simulink model "Model_14Bus_Microgrid_paper_Latam"  (R2022b)
settings: Solver=VariableStepAuto  StartTime=0.0  StopTime=0.5  MaxStep=1e-2  RelTol=1e-3
InitFcn:
  | Set_parameters_R2018
StopFcn:
  | %Save_Data;
  | %Graphics_mod;
values from neighbouring files (symbols this model uses):
  Clink = Ceq*2    (= 0.217013888889)    [Set_parameters.m]
  dis1 = 0.15    [Set_parameters.m]
  dis10 = 6    [Set_parameters.m]
  dis11 = 3    [Set_parameters.m]
  dis12 = 6    [Set_parameters.m]
  dis13 = 3    [Set_parameters.m]
  dis14 = 2    [Set_parameters.m]
  dis2 = 0.2    [Set_parameters.m]
  dis3 = 0.15    [Set_parameters.m]
  dis4 = 0.4    [Set_parameters.m]
  dis5 = 0.4    [Set_parameters.m]
  dis6 = 0.4    [Set_parameters.m]
  dis7 = 0.1    [Set_parameters.m]
  dis8 = 2    [Set_parameters.m]
  dis9 = 6    [Set_parameters.m]
  Fc = 33 * Fnom    (= 1980)    [Set_parameters.m]
  Fnom = 60    [Set_parameters.m]
  Increment_MPPT = 0.01    [Set_parameters.m]
  Ki_Ireg = 20    [Set_parameters.m]
  Ki_VDCreg = 400    [Set_parameters.m]
  Kp_Ireg = 0.3    [Set_parameters.m]
  Kp_VDCreg = 2    [Set_parameters.m]
  LimitL_Ireg = -1.5    [Set_parameters.m]
  LimitL_VDCreg = -1.5    [Set_parameters.m]
  Limits_MPPT = [ 583 357 ]    [Set_parameters.m]
  LimitU_Ireg = 1.5    [Set_parameters.m]
  LimitU_VDCreg = 1.5    [Set_parameters.m]
  P_Load_2 = S_Load_2* PF_Load_2    (= 36000)    [Set_parameters.m]
  P_Load_3 = S_Load_3* PF_Load_3    (= 25500)    [Set_parameters.m]
  Pnom = 1e6    (= 1000000)    [Set_parameters.m]
  Pnom_T1 = 1.5e6    (= 1500000)    [Set_parameters.m]
  Pnom_T2 = 1.5e6    (= 1500000)    [Set_parameters.m]
  Pnom_T3 = 4e6    (= 4000000)    [Set_parameters.m]
  Pnom_xfo = Pnom    (= 1000000)    [Set_parameters.m]
  Ql_Load_2 = S_Load_2 * sin(acos(PF_Load_2))    [Set_parameters.m]
  Ql_Load_3 = S_Load_3 * sin(acos(PF_Load_3))    [Set_parameters.m]
  R_Load_9 = (Vnom_prim * 1.35)^2 / P_Load_9    (= 1084.6153125)    [Set_parameters.m]
  R_Load_DC = Vnom_DC^2/ P_Load_DC    (= 45)    [Set_parameters.m]
  Rl = 0.394    [Set_parameters.m]
  Rls = 0.198    [Set_parameters.m]
  Ts = Ts_Power    (= 5.05050505051e-06)    [Set_parameters.m]
  Ts_Control = 10*Ts_Power    (= 5.05050505051e-05)    [Set_parameters.m]
  Ts_Power = 1/(33*Fnom)/100    (= 5.05050505051e-06)    [Set_parameters.m]
  V1_LL_T3 = 69e3    (= 69000)    [Set_parameters.m]
  Vf = 0    [Set_parameters.m]
  Vfd = 0    [Set_parameters.m]
  Vnom_dc = 480    [Set_parameters.m]
  Vnom_Diesel = 2.4e3    (= 2400)    [Set_parameters.m]
  Vnom_prim = 13.8e3    (= 13800)    [Set_parameters.m]
  Vnom_sec = 220    [Set_parameters.m]
  Vnom_ter_AC_DC = 150    [Set_parameters.m]
  Xl = 0.1168    [Set_parameters.m]
  Xls = 0.1089    [Set_parameters.m]
undefined symbols (not defined in the file or in its folder): D1, Delta, DiscIntNeverNeededParam, Hydride, Ion, level, Lithium, max_min, Metal, Nickel, RL, RLff, sigbuilder_block
libraries: spsRMSLib x73, powerlib_extras x53, spsCurrentMeasurementLib x47, spsTHDLib x26, spsThreePhaseVIMeasurementLib x25, spsVoltageMeasurementLib x23, spsSeriesRLCBranchLib x21, spsThreePhaseSeriesRLCBranchLib x21, spsIGBTDiodeLib x15, spsThreePhaseBreakerLib x14, spsPowerLib x14, spsThreePhaseTransformerTwoWindingsLib x12
(part 1 of 10)
settings Model: Creator=Leony  LastModifiedBy=christian
settings SolverCC: ZeroCrossAlgorithm=Adaptive  AlgebraicLoopSolver=TrustRegion  SolverResetMethod=Robust
settings DataIOCC: LimitDataPoints=on  SaveFormat=Array  ReturnWorkspaceOutputs=off
settings OptimizationCC: LifeSpan=inf  AccelVerboseBuild=on
settings DebuggingCC: AlgebraicLoopMsg=none  UnderspecifiedInitializationDetection=Classic  MergeDetectMultiDrivingBlocksExec=none  IgnoredZcDiagnostic=none  SolverPrmCheckMsg=warning  AllowSymbolicDim=off  SFUnexpectedBacktrackingDiag=warning  SFNoUnconditionalDefaultTransitionDiag=warning  SFExecutionAtInitializationDiag=none  SFMachineParentedDataDiag=warning  ArithmeticOperatorsInVariantConditions=warning
settings HardwareCC: ProdBitPerPointer=32  ProdBitPerSizeT=32  ProdBitPerPtrDiffT=32  ProdLargestAtomicFloat=None  ProdIntDivRoundTo=Undefined  ProdEndianess=Unspecified  ProdWordSize=32  ProdHWDeviceType=32-bit Generic
settings ModelReferenceCC: EnableRefExpFcnMdlSchedulingChecks=on  PropagateSignalLabelsOutOfModel=off
settings SFSimCC: SimUseLocalCustomCode=off  CustomCodeUndefinedFunction=UseInterfaceOnly
settings RTWCC: RTWUseLocalCustomCode=off  DLArmComputeVersion=19.05
settings CodeAppCC: StateflowObjectComments=on
settings GRTTargetCC: TargetLangStandard=C89/C90 (ANSI)
settings ConfigComp: CovMetricSettings=dw  CovSaveCumulativeToWorkspaceVar=on  CovSaveSingleToWorkspaceVar=on  CovExternalEMLEnable=off
settings SimscapeCC: SimscapeNormalizeSystem=off

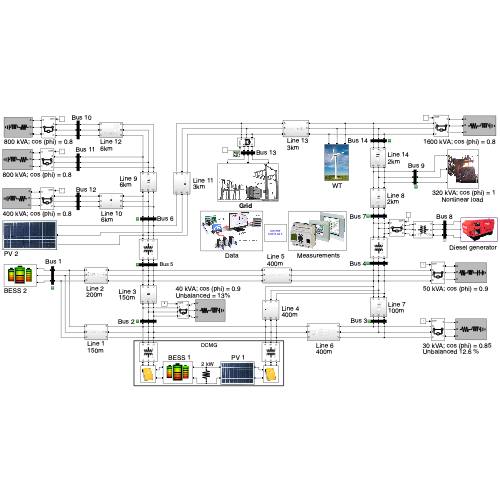
[thumbnail: Simulink's stored preview of the top-level diagram]
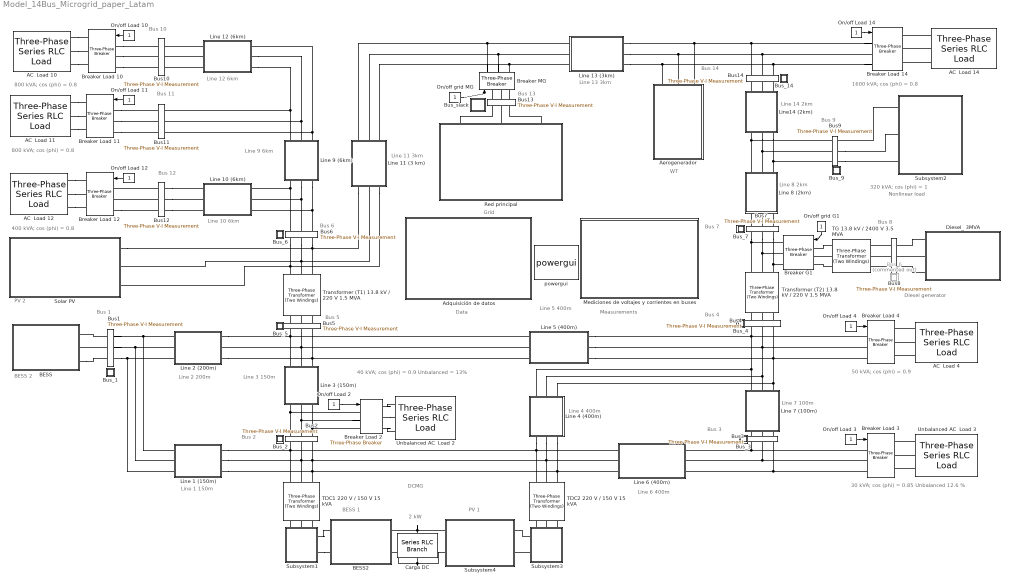
== system Model_14Bus_Microgrid_paper_Latam ==
  note: 1600 kVA; cos (phi) = 0.8
  note: 800 kVA; cos (phi) = 0.8
  note: 400 kVA; cos (phi) = 0.8
  note: 800 kVA; cos (phi) = 0.8
  note: 50 kVA; cos (phi) = 0.9
  note: 40 kVA; cos (phi) = 0.9
      | Unbalanced = 13%
  note: 2 kW
  note: 30 kVA; cos (phi) = 0.85
      | Unbalanced 12.6 %
  note: 320 kVA; cos (phi) = 1
  note: Diesel generator
  note: Line 7
      | 100m
  note: Bus 3
  note: Bus 2
  note: Bus 1
  note: Bus 5
  note: Bus 4
  note: Bus 6
  note: Bus 7
  note: Bus 9
  note: Bus 14
  note: Bus 8
  note: Line 8
      | 2km
  note: WT
  note: Line 13
      | 3km
  note: Line 14
      | 2km
  note: Bus 13
  note: Line 11
      | 3km
  note: Line 9
      | 6km
  note: Line 10
      | 6km
  note: Bus 12
  note: Bus 11
  note: Bus 10
  note: Line 12
      | 6km
  note: PV 2
  note: BESS 2
  note: Line 2
      | 200m
  note: Line 3
      | 150m
  note: Line 1
      | 150m
  note: Line 6
      | 400m
  note: Line 4
      | 400m
  note: Line 5
      | 400m
  note: BESS 1
  note: PV 1
  note: Grid
  note: Data
  note: Measurements
  note: Nonlinear load
  note: DCMG
  " Bus13" : spsThreePhaseVIMeasurementLib/Three-Phase V-I Measurement  VoltageMeasurement=phase-to-ground  SetLabelV=on  LabelV=Vabc_Sec  Vpu=off  VpuLL=off  CurrentMeasurement=yes  SetLabelI=on  LabelI=Iabc_Sec  Ipu=off  Pbase=100e6  Vbase=500e3  OutputType=Complex  PhasorSimulation=off  PSBequivalent=0
  AC  Load 10 : spsThreePhaseSeriesRLCLoadLib/Three-Phase Series RLC Load  LConnTagsString=A|B|C  Configuration=Y (grounded)  NominalVoltage=Vnom_prim  Vabc=[1e3 1e3 1e3]  Vabcp=[1e3 1e3 1e3]  NominalFrequency=Fnom  UnbalancedPower=off  ActivePower=P_Load_10  InductivePower=Ql_Load_10  CapacitivePower=0  Pabc=[10e3 9e3 11e3]  QLabc=[100 90 110]  QCabc=[100 90 110]  Pabcp=[10e3 9e3 11e3]  QLabcp=[100 90 110]  QCabcp=[100 90 110]  Measurements=None  LoadType=constant Z
  AC  Load 11 : spsThreePhaseSeriesRLCLoadLib/Three-Phase Series RLC Load  LConnTagsString=A|B|C  Configuration=Y (grounded)  NominalVoltage=Vnom_prim  Vabc=[1e3 1e3 1e3]  Vabcp=[1e3 1e3 1e3]  NominalFrequency=Fnom  UnbalancedPower=off  ActivePower=P_Load_11  InductivePower=Ql_Load_11  CapacitivePower=0  Pabc=[10e3 9e3 11e3]  QLabc=[100 90 110]  QCabc=[100 90 110]  Pabcp=[10e3 9e3 11e3]  QLabcp=[100 90 110]  QCabcp=[100 90 110]  Measurements=None  LoadType=constant Z
  AC  Load 12 : spsThreePhaseSeriesRLCLoadLib/Three-Phase Series RLC Load  LConnTagsString=A|B|C  Configuration=Y (grounded)  NominalVoltage=Vnom_prim  Vabc=[1e3 1e3 1e3]  Vabcp=[1e3 1e3 1e3]  NominalFrequency=Fnom  UnbalancedPower=off  ActivePower=P_Load_12  InductivePower=Ql_Load_12  CapacitivePower=0  Pabc=[10e3 9e3 11e3]  QLabc=[100 90 110]  QCabc=[100 90 110]  Pabcp=[10e3 9e3 11e3]  QLabcp=[100 90 110]  QCabcp=[100 90 110]  Measurements=None  LoadType=constant Z
  AC  Load 14 : spsThreePhaseSeriesRLCLoadLib/Three-Phase Series RLC Load  LConnTagsString=A|B|C  Configuration=Y (grounded)  NominalVoltage=Vnom_prim  Vabc=[1e3 1e3 1e3]  Vabcp=[1e3 1e3 1e3]  NominalFrequency=Fnom  UnbalancedPower=off  ActivePower=P_Load_14  InductivePower=Ql_Load_14  CapacitivePower=0  Pabc=[10e3 9e3 11e3]  QLabc=[100 90 110]  QCabc=[100 90 110]  Pabcp=[10e3 9e3 11e3]  QLabcp=[100 90 110]  QCabcp=[100 90 110]  Measurements=None  LoadType=constant Z
  AC  Load 4 : spsThreePhaseSeriesRLCLoadLib/Three-Phase Series RLC Load  LConnTagsString=A|B|C  Configuration=Y (grounded)  NominalVoltage=Vnom_sec  Vabc=[1e3 1e3 1e3]  Vabcp=[1e3 1e3 1e3]  NominalFrequency=Fnom  UnbalancedPower=on  ActivePower=P_Load_4  InductivePower=Ql_Load_4  CapacitivePower=0  Pabc=[10e3 9e3 11e3]  QLabc=[100 90 110]  QCabc=[100 90 110]  Pabcp=[10e3 9e3 11e3]  QLabcp=[100 90 110]  QCabcp=[100 90 110]  Measurements=None  LoadType=constant Z
  Adquisición de datos : Subsystem
      mask Display: image('/Users/christian/Documents/MATLAB/doctorado/4 conectada a la red con generador diesel, con generacion renovanble (fv)-con almacenamiento varios scope/Icons/SCADA.png'); % Use "Edit Image" on toolstrip to change.
  Aerogenerador : Subsystem
      settings: PortSchema="{\"entries\":[{\"content\":{\"sides\":[{\"content\":{\"connectorIds\":[]},\"type\":\"ConnectorPlacement.EquallySpacedRectSide\",\"uuid\":\"8edb4f72-423a-4d55-86f9-948b81889929\"},{\"content\":{\"connectorIds\":[],\"side\":\"RIGHT\"},\"type\":\"ConnectorPlacement.EquallySpacedRectSide\",\"uuid\":\"0da3ab69-be4e-4974-81d1-ba53ed348584\"},{\"content\":{\"connectorIds\":[\"LConn1\",\"LConn2\",\"LConn3\"],\"side\":\"TOP\"},\"type\":\"ConnectorPlacement.EquallySpacedRectSide\",\"uuid\":\"4000a557-50d9-4ea4-8b49-02707370a143\"}]},\"type\":\"ConnectorPlacement.EquallySpacedConnector\",\"uuid\":\"8a6f3a0d-9558-4751-993e-b03b26ac4eed\"}],\"packageUris\":[\"http://schema.mathworks.com/mf0/Connector/R2020b\"],\"version\":\"1.0\"}"
      mask Display: image('/Users/christian/Documents/MATLAB/doctorado/4 conectada a la red con generador diesel, con generacion renovanble (fv)-con almacenamiento varios scope/Icons/aerogenerador.jpeg'); % Use "Edit Image" on toolstrip to change.
  BESS : Subsystem
      mask Display: image('/Users/christian/Documents/MATLAB/doctorado/4 conectada a la red con generador diesel, con generacion renovanble (fv)-con almacenamiento varios scope/Icons/Battery Energy Storage System (BESS).png'); % Use "Edit Image" on toolstrip to change.
  BESS2 : Subsystem
      mask Display: image('/Users/christian/Documents/MATLAB/doctorado/4 conectada a la red con generador diesel, con generacion renovanble (fv)-con almacenamiento varios scope/Icons/Battery Energy Storage System (BESS).png'); % Use "Edit Image" on toolstrip to change.
  Breaker G1 : spsThreePhaseBreakerLib/Three-Phase Breaker  InitialState=closed  SwitchA=on  SwitchB=on  SwitchC=on  SwitchTimes="[4/60  10/60]"  External=on  BreakerResistance=0.001  SnubberResistance=1e6  SnubberCapacitance=inf  Measurements=None
  Breaker Load {2..4,10..12,14} (7 alike) : spsThreePhaseBreakerLib/Three-Phase Breaker  InitialState=closed  SwitchA=on  SwitchB=on  SwitchC=on  SwitchTimes="[4/60  10/60]"  External=on  BreakerResistance=0.001  SnubberResistance=1e6  SnubberCapacitance=inf  Measurements=None
  Breaker MG : spsThreePhaseBreakerLib/Three-Phase Breaker  InitialState=closed  SwitchA=on  SwitchB=on  SwitchC=on  SwitchTimes="[4/60  10/60]"  External=on  BreakerResistance=0.001  SnubberResistance=1e6  SnubberCapacitance=inf  Measurements=None
  Bus1 : spsThreePhaseVIMeasurementLib/Three-Phase V-I Measurement  VoltageMeasurement=phase-to-ground  SetLabelV=on  LabelV=VabcLL_Bus_1  Vpu=off  VpuLL=off  CurrentMeasurement=yes  SetLabelI=on  LabelI=IabcLL_Bus_1  Ipu=off  Pbase=100e6  Vbase=380/sqrt(2)  OutputType=Complex  PhasorSimulation=off  PSBequivalent=0
  Bus10 : spsThreePhaseVIMeasurementLib/Three-Phase V-I Measurement  VoltageMeasurement=phase-to-ground  SetLabelV=on  LabelV=VabcLL_Bus_10  Vpu=off  VpuLL=off  CurrentMeasurement=yes  SetLabelI=on  LabelI=IabcLL_Bus_10  Ipu=off  Pbase=100e6  Vbase=25e3/sqrt(2)  OutputType=Complex  PhasorSimulation=off  PSBequivalent=0
  Bus11 : spsThreePhaseVIMeasurementLib/Three-Phase V-I Measurement  VoltageMeasurement=phase-to-ground  SetLabelV=on  LabelV=VabcLL_Bus_11  Vpu=off  VpuLL=off  CurrentMeasurement=yes  SetLabelI=on  LabelI=IabcLL_Bus_11  Ipu=off  Pbase=100e6  Vbase=25e3/sqrt(2)  OutputType=Complex  PhasorSimulation=off  PSBequivalent=0
  Bus12 : spsThreePhaseVIMeasurementLib/Three-Phase V-I Measurement  VoltageMeasurement=phase-to-ground  SetLabelV=on  LabelV=VabcLL_Bus_12  Vpu=off  VpuLL=off  CurrentMeasurement=yes  SetLabelI=on  LabelI=IabcLL_Bus_12  Ipu=off  Pbase=100e6  Vbase=25e3  OutputType=Complex  PhasorSimulation=off  PSBequivalent=0
  Bus14 : spsThreePhaseVIMeasurementLib/Three-Phase V-I Measurement  VoltageMeasurement=phase-to-ground  SetLabelV=on  LabelV=VabcLL_Bus_14  Vpu=off  VpuLL=off  CurrentMeasurement=yes  SetLabelI=on  LabelI=IabcLL_Bus_14  Ipu=off  Pbase=100e6  Vbase=25e3/sqrt(2)  OutputType=Complex  PhasorSimulation=off  PSBequivalent=0
  Bus2 : spsThreePhaseVIMeasurementLib/Three-Phase V-I Measurement  VoltageMeasurement=phase-to-ground  SetLabelV=on  LabelV=VabcLL_Bus_2  Vpu=off  VpuLL=off  CurrentMeasurement=yes  SetLabelI=on  LabelI=IabcLL_Bus_2  Ipu=off  Pbase=100e6  Vbase=380/sqrt(2)  OutputType=Complex  PhasorSimulation=off  PSBequivalent=0
  Bus3 : spsThreePhaseVIMeasurementLib/Three-Phase V-I Measurement  VoltageMeasurement=phase-to-ground  SetLabelV=on  LabelV=VabcLL_Bus_3  Vpu=off  VpuLL=off  CurrentMeasurement=yes  SetLabelI=on  LabelI=IabcLL_Bus_3  Ipu=off  Pbase=100e6  Vbase=500e3  OutputType=Complex  PhasorSimulation=off  PSBequivalent=0
  Bus4 : spsThreePhaseVIMeasurementLib/Three-Phase V-I Measurement  VoltageMeasurement=phase-to-ground  SetLabelV=on  LabelV=VabcLL_Bus_4  Vpu=off  VpuLL=off  CurrentMeasurement=yes  SetLabelI=on  LabelI=IabcLL_Bus_4  Ipu=off  Pbase=100e6  Vbase=380/sqrt(2)  OutputType=Complex  PhasorSimulation=off  PSBequivalent=0
  Bus5 : spsThreePhaseVIMeasurementLib/Three-Phase V-I Measurement  VoltageMeasurement=phase-to-ground  SetLabelV=on  LabelV=VabcLL_Bus_5  Vpu=off  VpuLL=off  CurrentMeasurement=yes  SetLabelI=on  LabelI=IabcLL_Bus_5  Ipu=off  Pbase=100e6  Vbase=380/sqrt(2)  OutputType=Complex  PhasorSimulation=off  PSBequivalent=0
  Bus6 : spsThreePhaseVIMeasurementLib/Three-Phase V-I Measurement  VoltageMeasurement=phase-to-ground  SetLabelV=on  LabelV=VabcLL_Bus_6  Vpu=off  VpuLL=off  CurrentMeasurement=yes  SetLabelI=on  LabelI=IabcLL_Bus_6  Ipu=off  Pbase=100e6  Vbase=25e3/sqrt (2)  OutputType=Complex  PhasorSimulation=off  PSBequivalent=0
  Bus7_ : spsThreePhaseVIMeasurementLib/Three-Phase V-I Measurement  VoltageMeasurement=phase-to-ground  SetLabelV=on  LabelV=VabcLL_Bus_7  Vpu=off  VpuLL=off  CurrentMeasurement=yes  SetLabelI=on  LabelI=IabcLL_Bus_7  Ipu=off  Pbase=100e6  Vbase=25e3/sqrt(2)  OutputType=Complex  PhasorSimulation=off  PSBequivalent=0
  Bus8 : spsThreePhaseVIMeasurementLib/Three-Phase V-I Measurement  VoltageMeasurement=phase-to-ground  SetLabelV=on  LabelV=VabcLL_Bus_8  Vpu=off  VpuLL=off  CurrentMeasurement=yes  SetLabelI=on  LabelI=IabcLL_Bus_8  Ipu=off  Pbase=100e6  Vbase=25e3/sqrt(2)  OutputType=Complex  PhasorSimulation=off  PSBequivalent=0
  Bus9 : spsThreePhaseVIMeasurementLib/Three-Phase V-I Measurement  VoltageMeasurement=phase-to-ground  SetLabelV=on  LabelV=VabcLL_Bus_9  Vpu=off  VpuLL=off  CurrentMeasurement=yes  SetLabelI=on  LabelI=IabcLL_Bus_9  Ipu=off  Pbase=100e6  Vbase=25e3/sqrt(2)  OutputType=Complex  PhasorSimulation=off  PSBequivalent=0
  Bus_1 : Subsystem
  "Bus_14 " : Subsystem
  Bus_2 : Subsystem
  Bus_3 : Subsystem
  Bus_4 : Subsystem
  Bus_5 : Subsystem
  Bus_6 : Subsystem  Commented=on
  "Bus_6 " : Subsystem
  Bus_7 : Subsystem
  Bus_9 : Subsystem
  "Bus_slack " : Subsystem
      mask Display: image('/Users/christian/Documents/MATLAB/doctorado/4 conectada a la red con generador diesel, con generacion renovanble (fv)-con almacenamiento varios scope/Icons/S_meeter.png'); % Use "Edit Image" on toolstrip to change.
  Carga DC : spsSeriesRLCBranchLib/Series RLC Branch  LConnTagsString=__new0  RConnTagsString=__new0  BranchType=R  Resistance=R_Load_DC  Inductance=1e-3  SetiL0=off  InitialCurrent=0  Capacitance=1e-6  Setx0=off  InitialVoltage=0  Measurements=None
  Diesel_ 3MVA : Subsystem
      mask Display: image('/Users/christian/Documents/MATLAB/doctorado/4 conectada a la red con generador diesel, con generacion renovanble (fv)-con almacenamiento varios scope/Icons/Diesel 50kW1.png'); % Use "Edit Image" on toolstrip to change.
  Line 1 (150m) : Subsystem
  Line 10 (6km) : Subsystem
  Line 11 (3 km) : Subsystem
      settings: PortSchema="{\"entries\":[{\"content\":{\"sides\":[{\"content\":{\"connectorIds\":[]},\"type\":\"ConnectorPlacement.EquallySpacedRectSide\",\"uuid\":\"3fa4ce47-0618-4a86-9949-124e037c381d\"},{\"content\":{\"connectorIds\":[],\"side\":\"RIGHT\"},\"type\":\"ConnectorPlacement.EquallySpacedRectSide\",\"uuid\":\"4c990012-2922-4197-b7d6-ead729d5df02\"},{\"content\":{\"connectorIds\":[\"LConn1\",\"LConn2\",\"LConn3\"],\"side\":\"TOP\"},\"type\":\"ConnectorPlacement.EquallySpacedRectSide\",\"uuid\":\"f109a3c0-de9a-4d3f-a290-9f26370a4006\"},{\"content\":{\"connectorIds\":[\"RConn1\",\"RConn2\",\"RConn3\"],\"side\":\"BOTTOM\"},\"type\":\"ConnectorPlacement.EquallySpacedRectSide\",\"uuid\":\"1fb432e2-5f2a-4114-8f85-27692b44d437\"}]},\"type\":\"ConnectorPlacement.EquallySpacedConnector\",\"uuid\":\"f36c3437-0e44-4c49-a4c5-a4fab3944a97\"}],\"packageUris\":[\"http://schema.mathworks.com/mf0/Connector/R2020b\"],\"version\":\"1.0\"}"
  Line 12 (6km) : Subsystem
  Line 13 (3km) : Subsystem
  Line 2 (200m) : Subsystem
  Line 3 (150m) : Subsystem
      settings: PortSchema="{\"entries\":[{\"content\":{\"sides\":[{\"content\":{\"connectorIds\":[]},\"type\":\"ConnectorPlacement.EquallySpacedRectSide\",\"uuid\":\"c99559a6-214c-4b54-8932-e60695b83c0f\"},{\"content\":{\"connectorIds\":[],\"side\":\"RIGHT\"},\"type\":\"ConnectorPlacement.EquallySpacedRectSide\",\"uuid\":\"616e1f13-f43f-43c8-955c-af48087f0acf\"},{\"content\":{\"connectorIds\":[\"LConn1\",\"LConn2\",\"LConn3\"],\"side\":\"TOP\"},\"type\":\"ConnectorPlacement.EquallySpacedRectSide\",\"uuid\":\"d8640b2f-0936-4e22-9041-9217a77e250d\"},{\"content\":{\"connectorIds\":[\"RConn1\",\"RConn2\",\"RConn3\"],\"side\":\"BOTTOM\"},\"type\":\"ConnectorPlacement.EquallySpacedRectSide\",\"uuid\":\"49018893-7aca-42bb-82e4-1a5647518f54\"}]},\"type\":\"ConnectorPlacement.EquallySpacedConnector\",\"uuid\":\"7a3e400d-c0e2-4cae-aa4e-274e50cc0dcd\"}],\"packageUris\":[\"http://schema.mathworks.com/mf0/Connector/R2020b\"],\"version\":\"1.0\"}"
  Line 4 (400m) : Subsystem
      settings: PortSchema="{\"entries\":[{\"content\":{\"sides\":[{\"content\":{\"connectorIds\":[]},\"type\":\"ConnectorPlacement.EquallySpacedRectSide\",\"uuid\":\"c99559a6-214c-4b54-8932-e60695b83c0f\"},{\"content\":{\"connectorIds\":[],\"side\":\"RIGHT\"},\"type\":\"ConnectorPlacement.EquallySpacedRectSide\",\"uuid\":\"616e1f13-f43f-43c8-955c-af48087f0acf\"},{\"content\":{\"connectorIds\":[\"LConn1\",\"LConn2\",\"LConn3\"],\"side\":\"TOP\"},\"type\":\"ConnectorPlacement.EquallySpacedRectSide\",\"uuid\":\"d8640b2f-0936-4e22-9041-9217a77e250d\"},{\"content\":{\"connectorIds\":[\"RConn1\",\"RConn2\",\"RConn3\"],\"side\":\"BOTTOM\"},\"type\":\"ConnectorPlacement.EquallySpacedRectSide\",\"uuid\":\"d280c52d-8e8d-4714-b6e0-56518919c4ba\"}]},\"type\":\"ConnectorPlacement.EquallySpacedConnector\",\"uuid\":\"7a3e400d-c0e2-4cae-aa4e-274e50cc0dcd\"}],\"packageUris\":[\"http://schema.mathworks.com/mf0/Connector/R2020b\"],\"version\":\"1.0\"}"
  Line 5 (400m) : Subsystem
  Line 6 (400m) : Subsystem
  Line 7 (100m) : Subsystem
      settings: PortSchema="{\"entries\":[{\"content\":{\"sides\":[{\"content\":{\"connectorIds\":[]},\"type\":\"ConnectorPlacement.EquallySpacedRectSide\",\"uuid\":\"c99559a6-214c-4b54-8932-e60695b83c0f\"},{\"content\":{\"connectorIds\":[],\"side\":\"RIGHT\"},\"type\":\"ConnectorPlacement.EquallySpacedRectSide\",\"uuid\":\"616e1f13-f43f-43c8-955c-af48087f0acf\"},{\"content\":{\"connectorIds\":[\"LConn1\",\"LConn2\",\"LConn3\"],\"side\":\"TOP\"},\"type\":\"ConnectorPlacement.EquallySpacedRectSide\",\"uuid\":\"d8640b2f-0936-4e22-9041-9217a77e250d\"},{\"content\":{\"connectorIds\":[\"RConn1\",\"RConn2\",\"RConn3\"],\"side\":\"BOTTOM\"},\"type\":\"ConnectorPlacement.EquallySpacedRectSide\",\"uuid\":\"b0aa1ef5-75ce-4fbc-935e-e613957a7fe6\"}]},\"type\":\"ConnectorPlacement.EquallySpacedConnector\",\"uuid\":\"7a3e400d-c0e2-4cae-aa4e-274e50cc0dcd\"}],\"packageUris\":[\"http://schema.mathworks.com/mf0/Connector/R2020b\"],\"version\":\"1.0\"}"
  "Line 8 (2km) " : Subsystem
      settings: PortSchema="{\"entries\":[{\"content\":{\"sides\":[{\"content\":{\"connectorIds\":[]},\"type\":\"ConnectorPlacement.EquallySpacedRectSide\",\"uuid\":\"c99559a6-214c-4b54-8932-e60695b83c0f\"},{\"content\":{\"connectorIds\":[],\"side\":\"RIGHT\"},\"type\":\"ConnectorPlacement.EquallySpacedRectSide\",\"uuid\":\"616e1f13-f43f-43c8-955c-af48087f0acf\"},{\"content\":{\"connectorIds\":[\"LConn1\",\"LConn2\",\"LConn3\"],\"side\":\"TOP\"},\"type\":\"ConnectorPlacement.EquallySpacedRectSide\",\"uuid\":\"d8640b2f-0936-4e22-9041-9217a77e250d\"},{\"content\":{\"connectorIds\":[\"RConn1\",\"RConn2\",\"RConn3\"],\"side\":\"BOTTOM\"},\"type\":\"ConnectorPlacement.EquallySpacedRectSide\",\"uuid\":\"1877323f-0a18-4a2a-a644-81e35eb1883e\"}]},\"type\":\"ConnectorPlacement.EquallySpacedConnector\",\"uuid\":\"7a3e400d-c0e2-4cae-aa4e-274e50cc0dcd\"}],\"packageUris\":[\"http://schema.mathworks.com/mf0/Connector/R2020b\"],\"version\":\"1.0\"}"
  Line 9 (6km) : Subsystem
      settings: PortSchema="{\"entries\":[{\"content\":{\"sides\":[{\"content\":{\"connectorIds\":[]},\"type\":\"ConnectorPlacement.EquallySpacedRectSide\",\"uuid\":\"3fa4ce47-0618-4a86-9949-124e037c381d\"},{\"content\":{\"connectorIds\":[],\"side\":\"RIGHT\"},\"type\":\"ConnectorPlacement.EquallySpacedRectSide\",\"uuid\":\"4c990012-2922-4197-b7d6-ead729d5df02\"},{\"content\":{\"connectorIds\":[\"LConn1\",\"LConn2\",\"LConn3\"],\"side\":\"TOP\"},\"type\":\"ConnectorPlacement.EquallySpacedRectSide\",\"uuid\":\"f109a3c0-de9a-4d3f-a290-9f26370a4006\"},{\"content\":{\"connectorIds\":[\"RConn1\",\"RConn2\",\"RConn3\"],\"side\":\"BOTTOM\"},\"type\":\"ConnectorPlacement.EquallySpacedRectSide\",\"uuid\":\"0e33dc47-f0db-4c64-b17e-5caee7b79e41\"}]},\"type\":\"ConnectorPlacement.EquallySpacedConnector\",\"uuid\":\"f36c3437-0e44-4c49-a4c5-a4fab3944a97\"}],\"packageUris\":[\"http://schema.mathworks.com/mf0/Connector/R2020b\"],\"version\":\"1.0\"}"
  Line14 (2km) : Subsystem
      settings: PortSchema="{\"entries\":[{\"content\":{\"sides\":[{\"content\":{\"connectorIds\":[]},\"type\":\"ConnectorPlacement.EquallySpacedRectSide\",\"uuid\":\"c99559a6-214c-4b54-8932-e60695b83c0f\"},{\"content\":{\"connectorIds\":[],\"side\":\"RIGHT\"},\"type\":\"ConnectorPlacement.EquallySpacedRectSide\",\"uuid\":\"616e1f13-f43f-43c8-955c-af48087f0acf\"},{\"content\":{\"connectorIds\":[\"LConn1\",\"LConn2\",\"LConn3\"],\"side\":\"TOP\"},\"type\":\"ConnectorPlacement.EquallySpacedRectSide\",\"uuid\":\"d8640b2f-0936-4e22-9041-9217a77e250d\"},{\"content\":{\"connectorIds\":[\"RConn1\",\"RConn2\",\"RConn3\"],\"side\":\"BOTTOM\"},\"type\":\"ConnectorPlacement.EquallySpacedRectSide\",\"uuid\":\"02a8d416-77ac-4c7f-84b8-7eeb819b2c16\"}]},\"type\":\"ConnectorPlacement.EquallySpacedConnector\",\"uuid\":\"7a3e400d-c0e2-4cae-aa4e-274e50cc0dcd\"}],\"packageUris\":[\"http://schema.mathworks.com/mf0/Connector/R2020b\"],\"version\":\"1.0\"}"
  Mediciones de voltajes y corrientes en buses : Subsystem
      mask Display: image('/Users/christian/Documents/MATLAB/doctorado/4 conectada a la red con generador diesel, con generacion renovanble (fv)-con almacenamiento varios scope/Icons/PLC.png'); % Use "Edit Image" on toolstrip to change.
  On/off Load {2..4,10..12,14} (7 alike) : Constant
  On/off grid G1 : Constant
  On/off grid MG : Constant
  Red principal : Subsystem
      mask Display: image('/Users/christian/Documents/MATLAB/doctorado/4 conectada a la red con generador diesel, con generacion renovanble (fv)-con almacenamiento varios scope/Icons/transmision2.png'); % Use "Edit Image" on toolstrip to change.
  "Solar PV " : Subsystem
      settings: PortSchema="{\"entries\":[{\"content\":{\"sides\":[{\"content\":{\"connectorIds\":[]},\"type\":\"ConnectorPlacement.EquallySpacedRectSide\",\"uuid\":\"14311cf1-4565-4557-a9e5-8d1dd9d8828a\"},{\"content\":{\"connectorIds\":[],\"side\":\"RIGHT\"},\"type\":\"ConnectorPlacement.EquallySpacedRectSide\",\"uuid\":\"58266117-c53f-4571-994e-a375db018b9b\"},{\"content\":{\"connectorIds\":[],\"side\":\"TOP\"},\"type\":\"ConnectorPlacement.EquallySpacedRectSide\",\"uuid\":\"cef5be70-8480-48ac-bc24-64e7c3014e45\"},{\"content\":{\"connectorIds\":[\"RConn1\",\"RConn2\",\"RConn3\"],\"side\":\"BOTTOM\"},\"type\":\"ConnectorPlacement.EquallySpacedRectSide\",\"uuid\":\"d702a9d7-8194-4f70-a9b8-063d3b0b328a\"}]},\"type\":\"ConnectorPlacement.EquallySpacedConnector\",\"uuid\":\"0f093dd0-16af-46ad-a94c-f1a416e1fb10\"}],\"packageUris\":[\"http://schema.mathworks.com/mf0/Connector/R2020b\"],\"version\":\"1.0\"}"
      mask Display: image('/Users/christian/Documents/MATLAB/doctorado/4 conectada a la red con generador diesel, con generacion renovanble (fv)-con almacenamiento varios scope/Icons/PV.png'); % Use "Edit Image" on toolstrip to change.
  Subsystem1 : Subsystem
      settings: PortSchema="{\"entries\":[{\"content\":{\"sides\":[{\"content\":{\"connectorIds\":[\"LConn1\",\"LConn2\",\"LConn3\"]},\"type\":\"ConnectorPlacement.EquallySpacedRectSide\",\"uuid\":\"b2a5a210-a5c0-4a00-9ffb-bb6fdd4d112e\"},{\"content\":{\"connectorIds\":[],\"side\":\"RIGHT\"},\"type\":\"ConnectorPlacement.EquallySpacedRectSide\",\"uuid\":\"640eb224-e09d-4ff2-a9a2-97d7ca66d32e\"},{\"content\":{\"connectorIds\":[],\"side\":\"TOP\"},\"type\":\"ConnectorPlacement.EquallySpacedRectSide\",\"uuid\":\"1966b25b-a01e-4a3f-b0fd-7725ee45384c\"},{\"content\":{\"connectorIds\":[\"RConn1\",\"RConn2\"],\"side\":\"BOTTOM\"},\"type\":\"ConnectorPlacement.EquallySpacedRectSide\",\"uuid\":\"e9542c7a-ad47-42d1-807f-1d9756deacbb\"}]},\"type\":\"ConnectorPlacement.EquallySpacedConnector\",\"uuid\":\"6710c214-ed47-4514-bc2d-0db209adf1dd\"}],\"packageUris\":[\"http://schema.mathworks.com/mf0/Connector/R2020b\"],\"version\":\"1.0\"}"
      mask Display: image('/Users/christian/Documents/MATLAB/doctorado/4 conectada a la red con generador diesel, con generacion renovanble (fv)-con almacenamiento varios scope/Icons/Bi-directional converter.png'); % Use "Edit Image" on toolstrip to change.
  Subsystem2 : Subsystem
      mask Display: image('/Users/christian/Documents/MATLAB/doctorado/4 conectada a la red con generador diesel, con generacion renovanble (fv)-con almacenamiento varios scope/Icons/horno_de_arco.png'); % Use "Edit Image" on toolstrip to change.
  Subsystem3 : Subsystem
      settings: PortSchema="{\"entries\":[{\"content\":{\"sides\":[{\"content\":{\"connectorIds\":[\"LConn1\",\"LConn2\",\"LConn3\"]},\"type\":\"ConnectorPlacement.EquallySpacedRectSide\",\"uuid\":\"b2a5a210-a5c0-4a00-9ffb-bb6fdd4d112e\"},{\"content\":{\"connectorIds\":[],\"side\":\"RIGHT\"},\"type\":\"ConnectorPlacement.EquallySpacedRectSide\",\"uuid\":\"640eb224-e09d-4ff2-a9a2-97d7ca66d32e\"},{\"content\":{\"connectorIds\":[\"LConn4\",\"LConn5\"],\"side\":\"TOP\"},\"type\":\"ConnectorPlacement.EquallySpacedRectSide\",\"uuid\":\"1966b25b-a01e-4a3f-b0fd-7725ee45384c\"}]},\"type\":\"ConnectorPlacement.EquallySpacedConnector\",\"uuid\":\"6710c214-ed47-4514-bc2d-0db209adf1dd\"}],\"packageUris\":[\"http://schema.mathworks.com/mf0/Connector/R2020b\"],\"version\":\"1.0\"}"
      mask Display: image('/Users/christian/Documents/MATLAB/doctorado/4 conectada a la red con generador diesel, con generacion renovanble (fv)-con almacenamiento varios scope/Icons/Bi-directional converter.png'); % Use "Edit Image" on toolstrip to change.
  Subsystem4 : Subsystem
      settings: PortSchema="{\"entries\":[{\"content\":{\"sides\":[{\"content\":{\"connectorIds\":[]},\"type\":\"ConnectorPlacement.EquallySpacedRectSide\",\"uuid\":\"7999bb93-cf65-441d-8cac-9bbbf2d3b913\"},{\"content\":{\"connectorIds\":[],\"side\":\"RIGHT\"},\"type\":\"ConnectorPlacement.EquallySpacedRectSide\",\"uuid\":\"608a2d31-8c11-4711-81e5-197d370b4fca\"},{\"content\":{\"connectorIds\":[\"LConn1\",\"LConn2\"],\"side\":\"TOP\"},\"type\":\"ConnectorPlacement.EquallySpacedRectSide\",\"uuid\":\"f5ed2c17-0fec-4317-bdd6-228ff2b4758a\"},{\"content\":{\"connectorIds\":[\"RConn1\",\"RConn2\"],\"side\":\"BOTTOM\"},\"type\":\"ConnectorPlacement.EquallySpacedRectSide\",\"uuid\":\"fedfdf96-4c5c-4344-895b-a65cba0c778d\"}]},\"type\":\"ConnectorPlacement.EquallySpacedConnector\",\"uuid\":\"37159778-2ce3-4ce3-982f-761cad9e4348\"}],\"packageUris\":[\"http://schema.mathworks.com/mf0/Connector/R2020b\"],\"version\":\"1.0\"}"
      mask Display: image('/Users/christian/Documents/MATLAB/doctorado/4 conectada a la red con generador diesel, con generacion renovanble (fv)-con almacenamiento varios scope/Icons/PV.png'); % Use "Edit Image" on toolstrip to change.
  TDC1 220 V / 150 V 15 kVA : spsThreePhaseTransformerTwoWindingsLib/Three-Phase Transformer (Two Windings)  Winding1Connection=Y  Winding2Connection=Y  CoreType=Three single-phase transformers  SetSaturation=off  Hysteresis=off  DataFile='hysteresis'  SetInitialFlux=off  Measurements=None  UNITS=pu  NominalPower=[15e3 , Fnom ]  Winding1=[Vnom_sec , 0.03/2 , 0.03/377]  Winding2=[Vnom_ter_AC_DC , 0.03/2 , 0.03/377]  Rm=500  Lm=500  L0=0.5  Saturation=[ 0,0 ; 0.0024,1.2 ; 1.0,1.52 ]  InitialFluxes=[ 0.8 , -0.8 , 0.7 ]  BreakLoop=off  DiscreteSolver=Trapezoidal iterative  DataType=off  TransfoNumber=1
  TDC2 220 V / 150 V 15 kVA : spsThreePhaseTransformerTwoWindingsLib/Three-Phase Transformer (Two Windings)  Winding1Connection=Y  Winding2Connection=Y  CoreType=Three single-phase transformers  SetSaturation=off  Hysteresis=off  DataFile='hysteresis'  SetInitialFlux=off  Measurements=None  UNITS=pu  NominalPower=[15e3 , Fnom ]  Winding1=[Vnom_sec , 0.03/2 , 0.03/377 ]  Winding2=[Vnom_ter_AC_DC , 0.03/2 , 0.03/377 ]  Rm=500  Lm=500  L0=0.5  Saturation=[ 0,0 ; 0.0024,1.2 ; 1.0,1.52 ]  InitialFluxes=[ 0.8 , -0.8 , 0.7 ]  BreakLoop=off  DiscreteSolver=Trapezoidal iterative  DataType=off  TransfoNumber=1
  TG 13.8 kV / 2400 V 3.5 MVA : spsThreePhaseTransformerTwoWindingsLib/Three-Phase Transformer (Two Windings)  Winding1Connection=Yg  Winding2Connection=Delta (D1)  CoreType=Three single-phase transformers  SetSaturation=off  Hysteresis=off  DataFile='hysteresis'  SetInitialFlux=off  Measurements=None  UNITS=pu  NominalPower=[3.5e6 , Fnom ]  Winding1=[ Vnom_prim , 0.015/2 , 0.015/2/377]  Winding2=[ Vnom_Diesel , 0.015/2 , 0.015/2/377]  Rm=500  Lm=500  L0=0.5  Saturation="[ 0,0  ;  0.005,1.2  ;  1.0,1.4 ]"  InitialFluxes=[ 0.8 , -0.8 , 0.7 ]  BreakLoop=off  DiscreteSolver=Trapezoidal iterative  DataType=off  TransfoNumber=0
  Transformer (T1) 13.8 kV / 220 V 1.5 MVA : spsThreePhaseTransformerTwoWindingsLib/Three-Phase Transformer (Two Windings)  Winding1Connection=Y  Winding2Connection=Y  CoreType=Three single-phase transformers  SetSaturation=off  Hysteresis=off  DataFile='hysteresis'  SetInitialFlux=off  Measurements=None  UNITS=pu  NominalPower=[ Pnom_T1, Fnom ]  Winding1=[Vnom_prim , 0.03/2 , 0.03/(2*377) ]  Winding2=[Vnom_sec , 0.03/2 , 0.03/(2*377) ]  Rm=500  Lm=500  L0=0.5  Saturation=[ 0,0 ; 0.0024,1.2 ; 1.0,1.52 ]  InitialFluxes=[ 0.8 , -0.8 , 0.7 ]  BreakLoop=off  DiscreteSolver=Trapezoidal iterative  DataType=off  TransfoNumber=1
  Transformer (T2) 13.8 kV / 220 V 1.5 MVA : spsThreePhaseTransformerTwoWindingsLib/Three-Phase Transformer (Two Windings)  Winding1Connection=Y  Winding2Connection=Y  CoreType=Three single-phase transformers  SetSaturation=off  Hysteresis=off  DataFile='hysteresis'  SetInitialFlux=off  Measurements=None  UNITS=pu  NominalPower=[Pnom_T2 , Fnom]  Winding1=[ Vnom_prim, 0.03/2 , 0.03/(2*377) ]  Winding2=[Vnom_sec , 0.03/2 , 0.03/(2*377) ]  Rm=500  Lm=500  L0=0.5  Saturation=[ 0,0 ; 0.0024,1.2 ; 1.0,1.52 ]  InitialFluxes=[ 0.8 , -0.8 , 0.7 ]  BreakLoop=off  DiscreteSolver=Trapezoidal iterative  DataType=off  TransfoNumber=1
  Unbalanced AC  Load 2 : spsThreePhaseSeriesRLCLoadLib/Three-Phase Series RLC Load  LConnTagsString=A|B|C  Configuration=Y (grounded)  NominalVoltage=Vnom_sec  Vabc=[Vnom_sec/sqrt(3), Vnom_sec/sqrt(3), Vnom_sec/sqrt(3)]  Vabcp=[1e3 1e3 1e3]  NominalFrequency=Fnom  UnbalancedPower=on  ActivePower=P_Load_2  InductivePower=Ql_Load_2  CapacitivePower=0  Pabc=[P_Load_2, P_Load_2*0.85, P_Load_2*1.05]  QLabc=[Ql_Load_2, Ql_Load_2*0.85, Ql_Load_2*1.05]  QCabc=[0 0 0]  Pabcp=[10e3 9e3 11e3]  QLabcp=[100 90 110]  QCabcp=[100 90 110]  Measurements=None  LoadType=constant PQ
  Unbalanced AC  Load 3 : spsThreePhaseSeriesRLCLoadLib/Three-Phase Series RLC Load  LConnTagsString=A|B|C  Configuration=Y (grounded)  NominalVoltage=Vnom_sec  Vabc=[Vnom_sec/sqrt(3), Vnom_sec/sqrt(3), Vnom_sec/sqrt(3)]  Vabcp=[1e3 1e3 1e3]  NominalFrequency=Fnom  UnbalancedPower=on  ActivePower=P_Load_3  InductivePower=Ql_Load_3  CapacitivePower=0  Pabc=[P_Load_3*1.04, P_Load_3, P_Load_3*0.9]  QLabc=[Ql_Load_3*1.04, Ql_Load_3, Ql_Load_3*0.9]  QCabc=[0 0 0]  Pabcp=[10e3 9e3 11e3]  QLabcp=[100 90 110]  QCabcp=[100 90 110]  Measurements=None  LoadType=constant Z
  powergui : spspowerguiLib/powergui  Priority=1  SimulationMode=Discrete  SampleTime=Ts_Power  frequency=60  Iterations=50  frequencyindice=0  Pbase=100e6  ErrMax=1e-4  UnitsV=kV  UnitsW=kW  buscounter=27  FunctionMessages=off  echomessages=off  EnableUseOfTLC=off  CurrentSourceSwitches=off  DisableSnubberDevices=off  DisableRonSwitches=off  DisableVfSwitches=off  DisplayEquations=off  AutomaticDiscreteSolvers=off  SolverType=Tustin  Interpol=off  ExternalGateDelay=off  methode=off  Ts=0  x0status=blocks  SPID=off  SwTol=0  HookPort=off  NonlinearTolerance=1e-4  nMaxIteration=100  ContinueOnMaxIteration=off  RestoreLinks=warning  ResistiveCurrentMeasurement=off  Frange=[0:2:500]  Ylog=off  Xlog=on  ShowGrid=off  save=off  variable=ZData  structure=ScopeData12  ZoomFFT=off  StartTime=0.4  cycles=1  DisplayStyle=1  fundamental=60  FreqAxis=on  MaxFrequency=3000  frequencyindicesteady=1  RmsSteady=1  display=off
  wires:
  On/off grid MG/1 -> Breaker MG/1
  On/off Load 12/1 -> Breaker Load 12/1
  On/off Load 11/1 -> Breaker Load 11/1
  On/off Load 10/1 -> Breaker Load 10/1
  On/off Load 14/1 -> Breaker Load 14/1
  On/off Load 4/1 -> Breaker Load 4/1
  On/off Load 2/1 -> Breaker Load 2/1
  On/off Load 3/1 -> Breaker Load 3/1
  On/off grid G1/1 -> Breaker G1/1
  connections:
  Bus1/RConn2 -- Line 2 (200m)/LConn2 -- Line 1 (150m)/LConn2
  Bus2/RConn3 -- Line 3 (150m)/RConn3 -- Breaker Load 2/LConn3
  Breaker Load 4/LConn1 -- Bus4/RConn1 -- Line 5 (400m)/RConn1 -- Line 4 (400m)/LConn1 -- Line 7 (100m)/LConn1
  Breaker Load 4/LConn2 -- Bus4/RConn2 -- Line 7 (100m)/LConn2 -- Line 4 (400m)/LConn2 -- Line 5 (400m)/RConn2
  Breaker Load 4/LConn3 -- Bus4/RConn3 -- Line 5 (400m)/RConn3 -- Line 4 (400m)/LConn3 -- Line 7 (100m)/LConn3
  Line 3 (150m)/LConn1 -- Line 2 (200m)/RConn1 -- Line 5 (400m)/LConn1 -- Bus5/RConn1
  Breaker Load 3/LConn1 -- Bus3/RConn1 -- Line 6 (400m)/RConn1
  Breaker Load 3/LConn2 -- Bus3/RConn2 -- Line 6 (400m)/RConn2
  Breaker Load 3/LConn3 -- Bus3/RConn3 -- Line 6 (400m)/RConn3
  Bus6/LConn3 -- Transformer (T1) 13.8 kV / 220 V 1.5 MVA/LConn3 -- Line 11 (3 km)/RConn1 -- "Solar PV "/RConn3
  Line 12 (6km)/LConn3 -- Line 9 (6km)/LConn1 -- Bus11/LConn1
  Breaker MG/RConn1 -- Line 11 (3 km)/LConn1 -- Line 13 (3km)/LConn1
  Transformer (T2) 13.8 kV / 220 V 1.5 MVA/RConn1 -- Bus4/LConn1
  Transformer (T2) 13.8 kV / 220 V 1.5 MVA/RConn2 -- Bus4/LConn2
  Transformer (T2) 13.8 kV / 220 V 1.5 MVA/RConn3 -- Bus4/LConn3
  Bus7_/LConn2 -- Transformer (T2) 13.8 kV / 220 V 1.5 MVA/LConn2 -- Breaker G1/RConn2
  Bus7_/LConn3 -- Transformer (T2) 13.8 kV / 220 V 1.5 MVA/LConn3 -- Breaker G1/RConn3
  Line 13 (3km)/RConn3 -- Bus14/LConn3 -- Breaker Load 14/LConn3 -- Aerogenerador/LConn3
  Line14 (2km)/LConn3 -- Bus14/RConn3
  TDC1 220 V / 150 V 15 kVA/LConn1 -- TDC2 220 V / 150 V 15 kVA/LConn1 -- Line 6 (400m)/LConn1 -- Line 4 (400m)/RConn1 -- Line 1 (150m)/RConn1 -- Bus2/LConn1
  " Bus13"/RConn3 -- Breaker MG/LConn3
  " Bus13"/RConn2 -- Breaker MG/LConn2
  " Bus13"/RConn1 -- Breaker MG/LConn1
  Breaker Load 2/RConn1 -- Unbalanced AC  Load 2/LConn1
  Breaker Load 2/RConn2 -- Unbalanced AC  Load 2/LConn2
  Breaker Load 2/RConn3 -- Unbalanced AC  Load 2/LConn3
  AC  Load 12/LConn1 -- Breaker Load 12/RConn1
  AC  Load 12/LConn2 -- Breaker Load 12/RConn2
  AC  Load 12/LConn3 -- Breaker Load 12/RConn3
  Breaker Load 11/LConn1 -- Bus11/RConn1
  Breaker Load 11/LConn2 -- Bus11/RConn2
  Breaker Load 11/LConn3 -- Bus11/RConn3
  Breaker Load 10/LConn1 -- Bus10/RConn1
  Breaker Load 10/LConn2 -- Bus10/RConn2
  Breaker Load 10/LConn3 -- Bus10/RConn3
  AC  Load 10/LConn3 -- Breaker Load 10/RConn3
  AC  Load 10/LConn2 -- Breaker Load 10/RConn2
  AC  Load 10/LConn1 -- Breaker Load 10/RConn1
  AC  Load 14/LConn1 -- Breaker Load 14/RConn1
  AC  Load 14/LConn2 -- Breaker Load 14/RConn2
  AC  Load 14/LConn3 -- Breaker Load 14/RConn3
  AC  Load 4/LConn1 -- Breaker Load 4/RConn1
  AC  Load 4/LConn2 -- Breaker Load 4/RConn2
  AC  Load 4/LConn3 -- Breaker Load 4/RConn3
  Bus12/RConn1 -- Breaker Load 12/LConn1
  Bus12/RConn2 -- Breaker Load 12/LConn2
  Breaker Load 12/LConn3 -- Bus12/RConn3
  Bus6/RConn3 -- Line 9 (6km)/RConn3 -- Line 10 (6km)/LConn3
  Bus6/RConn1 -- Line 9 (6km)/RConn1 -- Line 10 (6km)/LConn1
  Unbalanced AC  Load 3/LConn3 -- Breaker Load 3/RConn3
  Unbalanced AC  Load 3/LConn1 -- Breaker Load 3/RConn1
  Unbalanced AC  Load 3/LConn2 -- Breaker Load 3/RConn2
  Line 13 (3km)/RConn2 -- Bus14/LConn2 -- Breaker Load 14/LConn2 -- Aerogenerador/LConn2
  AC  Load 11/LConn1 -- Breaker Load 11/RConn1
  AC  Load 11/LConn2 -- Breaker Load 11/RConn2
  AC  Load 11/LConn3 -- Breaker Load 11/RConn3
  Bus1/LConn1 -- BESS/RConn1
  Bus1/LConn2 -- BESS/RConn2
  BESS/RConn3 -- Bus1/LConn3
  Transformer (T1) 13.8 kV / 220 V 1.5 MVA/LConn1 -- "Solar PV "/RConn1 -- Line 11 (3 km)/RConn3 -- Bus6/LConn1
  Line 11 (3 km)/RConn2 -- Transformer (T1) 13.8 kV / 220 V 1.5 MVA/LConn2 -- "Solar PV "/RConn2 -- Bus6/LConn2
  Red principal/LConn1 -- " Bus13"/LConn1
  Red principal/LConn3 -- " Bus13"/LConn3
  Red principal/LConn2 -- " Bus13"/LConn2
  TDC2 220 V / 150 V 15 kVA/RConn1 -- Subsystem3/LConn1
  TDC2 220 V / 150 V 15 kVA/RConn2 -- Subsystem3/LConn2
  TDC2 220 V / 150 V 15 kVA/RConn3 -- Subsystem3/LConn3
  TDC1 220 V / 150 V 15 kVA/RConn1 -- Subsystem1/LConn1
  TDC1 220 V / 150 V 15 kVA/RConn2 -- Subsystem1/LConn2
  TDC1 220 V / 150 V 15 kVA/RConn3 -- Subsystem1/LConn3
  Carga DC/RConn1 -- BESS2/RConn1 -- Subsystem4/LConn2
  Subsystem3/LConn4 -- Subsystem4/RConn2
  Subsystem3/LConn5 -- Subsystem4/RConn1
  Subsystem4/LConn1 -- Carga DC/LConn1 -- BESS2/RConn2
  Subsystem1/RConn2 -- BESS2/LConn2
  Subsystem1/RConn1 -- BESS2/LConn1
  Subsystem2/LConn1 -- Bus9/RConn1
  Bus9/RConn2 -- Subsystem2/LConn2
  Bus9/RConn3 -- Subsystem2/LConn3
  Line14 (2km)/RConn2 -- Bus9/LConn2 -- "Line 8 (2km) "/LConn2
  Line14 (2km)/RConn1 -- "Line 8 (2km) "/LConn1 -- Bus9/LConn1
  Bus9/LConn3 -- Line14 (2km)/RConn3 -- "Line 8 (2km) "/LConn3
  Bus3/LConn1 -- Line 7 (100m)/RConn1
  Bus3/LConn2 -- Line 7 (100m)/RConn2
  Bus3/LConn3 -- Line 7 (100m)/RConn3
  Bus1/RConn1 -- Line 2 (200m)/LConn1 -- Line 1 (150m)/LConn1
  Bus1/RConn3 -- Line 2 (200m)/LConn3 -- Line 1 (150m)/LConn3
  Line 3 (150m)/LConn3 -- Line 5 (400m)/LConn3 -- Line 2 (200m)/RConn3 -- Bus5/RConn3
  Line 3 (150m)/LConn2 -- Line 2 (200m)/RConn2 -- Line 5 (400m)/LConn2 -- Bus5/RConn2
  Breaker MG/RConn3 -- Line 11 (3 km)/LConn3 -- Line 13 (3km)/LConn3
  Breaker MG/RConn2 -- Line 11 (3 km)/LConn2 -- Line 13 (3km)/LConn2
  Line 12 (6km)/RConn1 -- Bus10/LConn1
  Line 12 (6km)/RConn2 -- Bus10/LConn2
  Line 12 (6km)/RConn3 -- Bus10/LConn3
  Bus6/RConn2 -- Line 9 (6km)/RConn2 -- Line 10 (6km)/LConn2
  Line 9 (6km)/LConn3 -- Line 12 (6km)/LConn1 -- Bus11/LConn3
  Line 12 (6km)/LConn2 -- Line 9 (6km)/LConn2 -- Bus11/LConn2
  Bus12/LConn1 -- Line 10 (6km)/RConn1
  Bus12/LConn2 -- Line 10 (6km)/RConn2
  Bus12/LConn3 -- Line 10 (6km)/RConn3
  Line14 (2km)/LConn2 -- Bus14/RConn2
  Bus8/RConn2 -- TG 13.8 kV / 2400 V 3.5 MVA/RConn2
  Diesel_ 3MVA/LConn3 -- Bus8/LConn3
  Bus8/RConn1 -- TG 13.8 kV / 2400 V 3.5 MVA/RConn1
  Bus7_/LConn1 -- Transformer (T2) 13.8 kV / 220 V 1.5 MVA/LConn1 -- Breaker G1/RConn1
  Diesel_ 3MVA/LConn1 -- Bus8/LConn1
  Diesel_ 3MVA/LConn2 -- Bus8/LConn2
  TG 13.8 kV / 2400 V 3.5 MVA/LConn1 -- Breaker G1/LConn1
  TG 13.8 kV / 2400 V 3.5 MVA/LConn2 -- Breaker G1/LConn2
  Bus8/RConn3 -- TG 13.8 kV / 2400 V 3.5 MVA/RConn3
  TG 13.8 kV / 2400 V 3.5 MVA/LConn3 -- Breaker G1/LConn3
  Bus2/RConn2 -- Line 3 (150m)/RConn2 -- Breaker Load 2/LConn2
  Bus7_/RConn1 -- "Line 8 (2km) "/RConn1
  Bus7_/RConn2 -- "Line 8 (2km) "/RConn2
  Bus7_/RConn3 -- "Line 8 (2km) "/RConn3
  TDC1 220 V / 150 V 15 kVA/LConn2 -- TDC1 220 V / 150 V 15 kVA/LConn3 -- TDC2 220 V / 150 V 15 kVA/LConn3 -- Line 6 (400m)/LConn3 -- Line 4 (400m)/RConn3 -- Line 1 (150m)/RConn3 -- Line 4 (400m)/RConn2 -- Line 6 (400m)/LConn2 -- TDC2 220 V / 150 V 15 kVA/LConn2 -- Bus2/LConn3 -- Bus2/LConn2 -- Line 1 (150m)/RConn2
  Bus2/RConn1 -- Line 3 (150m)/RConn1 -- Breaker Load 2/LConn1
  Transformer (T1) 13.8 kV / 220 V 1.5 MVA/RConn1 -- Bus5/LConn1
  Transformer (T1) 13.8 kV / 220 V 1.5 MVA/RConn3 -- Bus5/LConn3
  Transformer (T1) 13.8 kV / 220 V 1.5 MVA/RConn2 -- Bus5/LConn2
  Line14 (2km)/LConn1 -- Bus14/RConn1
  Line 13 (3km)/RConn1 -- Breaker Load 14/LConn1 -- Bus14/LConn1 -- Aerogenerador/LConn1

== system Model_14Bus_Microgrid_paper_Latam/Adquisición de datos ==
  note: Transformador (T1)
  note: Mediciones
  Delta_abc : Subsystem  Commented=on
  PF_abc : Subsystem
  P_abc : Subsystem
  Power_Losses_abc : Subsystem  Commented=on
  Q_abc : Subsystem
  RMS1 : spsRMSLib/RMS  TrueRMS=on  Freq=60  RMSInit=0  Ts=0
  RMS2 : spsRMSLib/RMS  TrueRMS=on  Freq=60  RMSInit=0  Ts=0
  THDi_abc : Subsystem
  THDv_abc : Subsystem
  VoltageLL_pu_abc : Subsystem
  scope 11 : Scope
  scope 12 : Scope
  wires:
  [Vabc_Sec_pu] -> RMS1/1
  RMS1/1 -> scope 11/1
  RMS2/1 -> scope 12/1
  [Vabc_Prim_pu] -> RMS2/1  "Signal Vabc"

== system Model_14Bus_Microgrid_paper_Latam/Aerogenerador ==
  B575 (575 V)1 : spsThreePhaseVIMeasurementLib/Three-Phase V-I Measurement  VoltageMeasurement=phase-to-ground  SetLabelV=on  LabelV=Vabc_B13kv  Vpu=off  VpuLL=off  CurrentMeasurement=yes  SetLabelI=on  LabelI=Iabc_B13kv  Ipu=off  Pbase=750e3%1.5e6  Vbase=575  OutputType=Complex  PhasorSimulation=off  PSBequivalent=0
  B575 (575 V)2 : spsThreePhaseVIMeasurementLib/Three-Phase V-I Measurement  VoltageMeasurement=phase-to-ground  SetLabelV=on  LabelV=Vabc_Aero  Vpu=off  VpuLL=off  CurrentMeasurement=yes  SetLabelI=on  LabelI=Iabc_Aero  Ipu=off  Pbase=750e3%1.5e6  Vbase=575  OutputType=Complex  PhasorSimulation=off  PSBequivalent=0
  B575 PU (575 V) : spsThreePhaseVIMeasurementLib/Three-Phase V-I Measurement  VoltageMeasurement=phase-to-ground  SetLabelV=on  LabelV=Vabc_B575  Vpu=on  VpuLL=off  CurrentMeasurement=yes  SetLabelI=on  LabelI=Iabc_B575  Ipu=on  Pbase=750e3%1.5e6  Vbase=575  OutputType=Complex  PhasorSimulation=off  PSBequivalent=0
  Breaker Load 1 : spsThreePhaseBreakerLib/Three-Phase Breaker  InitialState=closed  SwitchA=on  SwitchB=on  SwitchC=on  SwitchTimes="[4/60  10/60]"  External=on  BreakerResistance=0.001  SnubberResistance=1e6  SnubberCapacitance=inf  Measurements=None
  On/off Load 1 : Constant
  PMSG Wind Turbine1 : Subsystem  mask{Vnom=575, Pnom=0.75e6, Fnom=60, RL_grid=[0.003 0.3], Vdc_nom=1150, Np=48, Fb_time_const=0.005}
      mask prompts: Vnom "Rated L-L Voltage(V)"; Pnom "Rated Power(VA)"; Fnom "Rated Frequency(Hz)"; RL_grid "Grid-side coupling impedance(p.u.)"; Vdc_nom "DC capacitor voltage(V)"; Np "Number of pole pairs"; Fb_time_const "Feed back time constant(s)"
      mask init:
      | R_RL=RL_grid(1);
      | L_RL=RL_grid(2);
      mask Display: image('/Users/christian/Documents/MATLAB/doctorado/4 conectada a la red con generador diesel, con generacion renovanble (fv)-con almacenamiento varios scope/Icons/aerogenerador.jpeg'); % Use "Edit Image" on toolstrip to change.
  TB 575 V / 220 V 1.5 MVA2 : spsThreePhaseTransformerTwoWindingsLib/Three-Phase Transformer (Two Windings)  Commented=on  Winding1Connection=Delta (D1)  Winding2Connection=Yg  CoreType=Three single-phase transformers  SetSaturation=off  Hysteresis=off  DataFile='hysteresis'  SetInitialFlux=off  Measurements=None  UNITS=pu  NominalPower=[ 1.5e6 , Fnom ]  Winding1=[ 575 , 0.0015 , 0.03]  Winding2=[Vnom_sec , 0.03/2 , 0.03/(2*377) ]  Rm=200  Lm=200  L0=0.5  Saturation="[ 0,0  ;  0.005,1.2  ;  1.0,1.4 ]"  InitialFluxes=[ 0.8 , -0.8 , 0.7 ]  BreakLoop=off  DiscreteSolver=Trapezoidal iterative  DataType=off  TransfoNumber=0
  TB daian 575 V / 220 V 1.5 MVA1 : spsThreePhaseTransformerTwoWindingsLib/Three-Phase Transformer (Two Windings)  Commented=on  Winding1Connection=Delta (D1)  Winding2Connection=Yg  CoreType=Three single-phase transformers  SetSaturation=off  Hysteresis=off  DataFile='hysteresis'  SetInitialFlux=off  Measurements=None  UNITS=pu  NominalPower=[ 1.5e6 , Fnom ]  Winding1=[ 575 , 0.0012 , 0.03]  Winding2=[Vnom_sec, 0.0012, 0.0300]  Rm=200  Lm=200  L0=0.5  Saturation="[ 0,0  ;  0.005,1.2  ;  1.0,1.4 ]"  InitialFluxes=[ 0.8 , -0.8 , 0.7 ]  BreakLoop=off  DiscreteSolver=Trapezoidal iterative  DataType=off  TransfoNumber=0
  TG 13.8 kV / 575V : spsThreePhaseTransformerTwoWindingsLib/Three-Phase Transformer (Two Windings)  Commented=on  Winding1Connection=Yg  Winding2Connection=Delta (D1)  CoreType=Three single-phase transformers  SetSaturation=off  Hysteresis=off  DataFile='hysteresis'  SetInitialFlux=off  Measurements=None  UNITS=pu  NominalPower=[3.5e6 , Fnom ]  Winding1=[ Vnom_prim , 0.015/2 , 0.015/2/377]  Winding2=[ 575 , 0.015/2 , 0.015/2/377]  Rm=500  Lm=500  L0=0.5  Saturation="[ 0,0  ;  0.005,1.2  ;  1.0,1.4 ]"  InitialFluxes=[0.80001 -0.80001 0.7]  BreakLoop=off  DiscreteSolver=Trapezoidal iterative  DataType=off  TransfoNumber=0
  TG_damian 13.8 kV / 575V1 : spsThreePhaseTransformerTwoWindingsLib/Three-Phase Transformer (Two Windings)  Winding1Connection=Yg  Winding2Connection=Delta (D1)  CoreType=Three single-phase transformers  SetSaturation=off  Hysteresis=off  DataFile='hysteresis'  SetInitialFlux=off  Measurements=None  UNITS=pu  NominalPower=[3.5e6 , Fnom ]  Winding1=W1_xfo  Winding2=[ 575 , 0.0012, 0.0300]  Rm=200  Lm=200  L0=0.5  Saturation="[ 0,0  ;  0.005,1.2  ;  1.0,1.4 ]"  InitialFluxes=[0.80001 -0.80001 0.7]  BreakLoop=off  DiscreteSolver=Trapezoidal iterative  DataType=off  TransfoNumber=0
  A : PMIOPort  Side=Left
  B : PMIOPort  Port=2  Side=Left
  C : PMIOPort  Port=3  Side=Left
  wires:
  On/off Load 1/1 -> Breaker Load 1/1
  connections:
  B575 (575 V)1/LConn2 -- B/RConn1
  B575 (575 V)2/RConn1 -- B575 PU (575 V)/LConn1
  B575 (575 V)1/RConn3 -- Breaker Load 1/LConn3
  B575 (575 V)1/RConn2 -- Breaker Load 1/LConn2
  PMSG Wind Turbine1/RConn3 -- B575 PU (575 V)/RConn3
  PMSG Wind Turbine1/RConn1 -- B575 PU (575 V)/RConn1
  B575 (575 V)2/RConn2 -- B575 PU (575 V)/LConn2
  B575 (575 V)1/RConn1 -- Breaker Load 1/LConn1
  B575 PU (575 V)/LConn3 -- B575 (575 V)2/RConn3
  B575 (575 V)1/LConn1 -- A/RConn1
  B575 (575 V)1/LConn3 -- C/RConn1
  PMSG Wind Turbine1/RConn2 -- B575 PU (575 V)/RConn2
  TG_damian 13.8 kV / 575V1/LConn2 -- Breaker Load 1/RConn2
  TG_damian 13.8 kV / 575V1/LConn1 -- Breaker Load 1/RConn1
  TG_damian 13.8 kV / 575V1/LConn3 -- Breaker Load 1/RConn3
  TG_damian 13.8 kV / 575V1/RConn2 -- B575 (575 V)2/LConn2
  B575 (575 V)2/LConn3 -- TG_damian 13.8 kV / 575V1/RConn3
  TG_damian 13.8 kV / 575V1/RConn1 -- B575 (575 V)2/LConn1
